simulink model "OFDM_8_Point"  (R2022a)
settings: Solver=VariableStepAuto  StartTime=0.0  StopTime=1000  RelTol=1e-3
undefined symbols (not defined in the file): xc7s100fgga676
libraries: hdlBasic x39, commrandsrc3 x1, vmcUtilities x1
settings Model: Creator=Sandesh  LastModifiedBy=Sandesh

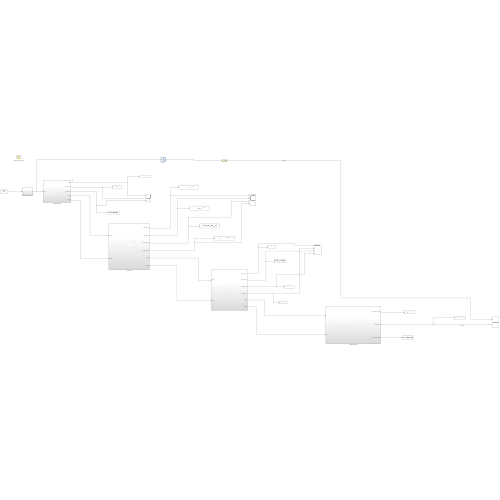
[thumbnail: Simulink's stored preview of the top-level diagram]
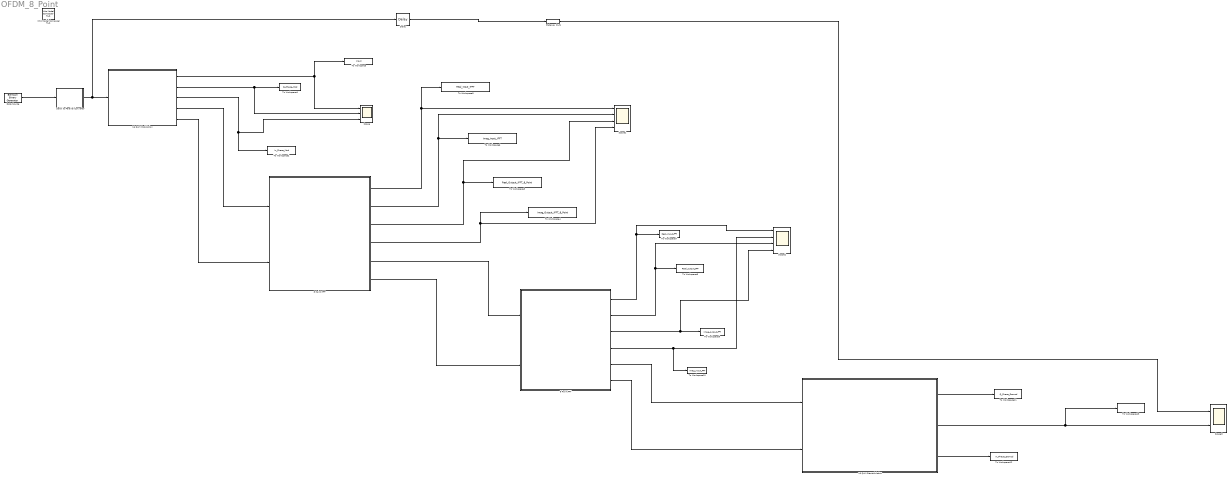
== system OFDM_8_Point ==
  16 QAM Demodulation : Subsystem
  16 QAM Modulation : Subsystem
  8 Point FFT : Subsystem
  8 Point IFFT : Subsystem
  Data Source : commrandsrc3/Bernoulli Binary Generator  ProbabilityOfZero=0.5  SeedSource=Auto  Seed=0  SampleTime=1  SamplesPerFrame=1  OutputDataType=double  SimulateUsing=Interpreted execution
  Delay : hdlBasic/Delay  rst=off  en=off  latency=129  reg_retiming=off  XmcBlockStatus=1  maskContainerNames=group1  block_type=delay  block_config=sysgen:Delay_config
  Gateway Out1 : hdlBasic/Gateway Out  inherit_from_input=off  hdl_port=on  rows=1  columns=1  UseAsDAC=off  DACChannel='1'  interface=None  automatic_assignment=on  address_offset=hex2dec('00')  intf_name=''  intf_description=''  timing_constraint=None  locs_specified=off  LOCs={}  io_standard={}  XmcBlockStatus=1  maskContainerNames=group4  block_type=gatewayout  block_config=sysgen:gateway_out_config  block_width_w=590  block_height_w=620  block_width=620  block_height=750
  Scope : Scope  NumInputPorts=3
  Scope1 : Scope  NumInputPorts=4
  Scope2 : Scope  NumInputPorts=4
  Scope3 : Scope  NumInputPorts=2
  Serial to Parallel Converter : Subsystem
  To Workspace : ToWorkspace  VariableName=Input  SaveFormat=Timeseries  SampleTime=-1
  To Workspace1 : ToWorkspace  VariableName=Q_Phase_Mod  SaveFormat=Timeseries  SampleTime=-1
  To Workspace10 : ToWorkspace  VariableName=Imag_Input_FFT  SaveFormat=Timeseries  SampleTime=-1
  To Workspace11 : ToWorkspace  VariableName=Q_Phase_Demod  SaveFormat=Timeseries  SampleTime=-1
  To Workspace12 : ToWorkspace  VariableName=In_Phase_Demod  SaveFormat=Timeseries  SampleTime=-1
  To Workspace13 : ToWorkspace  VariableName=Output_after_demodulation  SaveFormat=Timeseries  SampleTime=-1
  To Workspace2 : ToWorkspace  VariableName=In_Phase_Mod  SaveFormat=Timeseries  SampleTime=-1
  To Workspace3 : ToWorkspace  VariableName=Real_Output_IFFT_8_Point  SaveFormat=Timeseries  SampleTime=-1
  To Workspace4 : ToWorkspace  VariableName=Imag_Output_IFFT_8_Point  SaveFormat=Timeseries  SampleTime=-1
  To Workspace5 : ToWorkspace  VariableName=Real_Input_IFFT  SaveFormat=Timeseries  SampleTime=-1
  To Workspace6 : ToWorkspace  VariableName=Imag_Input_IFFT  SaveFormat=Timeseries  SampleTime=-1
  To Workspace7 : ToWorkspace  VariableName=Real_Input_FFT  SaveFormat=Timeseries  SampleTime=-1
  To Workspace8 : ToWorkspace  VariableName=Real_output_FFT  SaveFormat=Timeseries  SampleTime=-1
  To Workspace9 : ToWorkspace  VariableName=Imag_output_FFT  SaveFormat=Timeseries  SampleTime=-1
  Vitis Model Composer Hub : vmcUtilities/Vitis Model Composer Hub  Tag=genX  CodeGeneration=off  TargetDirectory=./code  ExportType=AI Engines  IpVendor=xilinx.com  IpLibrary=hls  IpVersion=1.0  IpHWLanguage=Verilog  AieCompilerOptions={}  CreateTestbench=off  TestbenchStackSize=10  RunAieSim=off  AieSimTimeout=50000  RunAieSimProfiling=off  LaunchVitisAnalyzer=off  PlotOutput=off  RunX86Sim=off  X86SimTimeout=10  GenHwImage=off  PlatformType=Not Specified  HwSystemType=Baremetal  HwValidationTarget=hw  ProjDevice=Spartan-7 SP701 Evaluation Platform (xc7s100fgga676-2)  ProjDevicePart=xc7s100fgga676-2  SamplePeriod=-1  ClockFrequency=200  DataPathParallelism=1  xilinxfamily=spartan7  part=xc7s100  speed=-2  package=fgga676  directory=./netlist  testbench=on  incr_netlist=off  synthesis_tool=Vivado  clock_wrapper=Clock Enables  dbl_ovrd=According to Block Masks  dcm_input_clock_period=10  sysclk_period=10  simulink_period=1  eval_field=0  IPInfoJsonString="{\"HDLSubsystem\":{\"SubsystemName\":\"QAM_16_Point\",\"IPName\":\"QAM_16_Point\",\"IPLibrary\":\"VMC\",\"IPVendor\":\"User Company\",\"IPVersion\":\"1.0\"}}"
  wires:
  Data Source/1 -> Serial to Parallel Converter/1(S)
  8 Point IFFT/4(Imag_Output_IFFT) -> Scope1/4, To Workspace4/1
  8 Point IFFT/3(Real_Output_IFFT) -> Scope1/3, To Workspace3/1
  8 Point IFFT/2(Imag_Input_IFFT) -> Scope1/2, To Workspace6/1
  8 Point IFFT/1(Real_Input_IFFT) -> Scope1/1, To Workspace5/1
  8 Point FFT/2(Real_Output_FFT) -> Scope2/3, To Workspace8/1
  8 Point FFT/3(Imag_Output_FFT) -> To Workspace9/1, Scope2/4
  8 Point FFT/1(Real_Input_FFT) -> Scope2/1, To Workspace7/1
  8 Point FFT/4(Imag_Input_FFT) -> Scope2/2, To Workspace10/1
  8 Point IFFT/5(Real_Out) -> 8 Point FFT/1(In_Real)
  8 Point IFFT/6(Imag_Out) -> 8 Point FFT/2(In_Imag)
  Delay/1 -> Gateway Out1/1
  Gateway Out1/1 -> Scope3/1  "Initial_Input"
  16 QAM Demodulation/2(DeMod_Output) -> Scope3/2, To Workspace13/1  "Final_Output"
  8 Point FFT/5(Imag_out) -> 16 QAM Demodulation/1(Q_Phase)
  8 Point FFT/6(Real_out) -> 16 QAM Demodulation/2(In_Phase)
  16 QAM Demodulation/1(Q_Phase_Dmod_Output) -> To Workspace11/1
  16 QAM Demodulation/3(In_Phase_Dmod_Output) -> To Workspace12/1
  Serial to Parallel Converter/1(P) -> 16 QAM Modulation/1(In_4_bit), Delay/1
  16 QAM Modulation/1(Input) -> Scope/1, To Workspace/1
  16 QAM Modulation/3(In_Phase_Mod1) -> Scope/3, To Workspace2/1
  16 QAM Modulation/2(Q_Phase_Mod1) -> Scope/2, To Workspace1/1
  16 QAM Modulation/4(Real_In) -> 8 Point IFFT/1(In_Real)
  16 QAM Modulation/5(Imag_In) -> 8 Point IFFT/2(In_Imag)

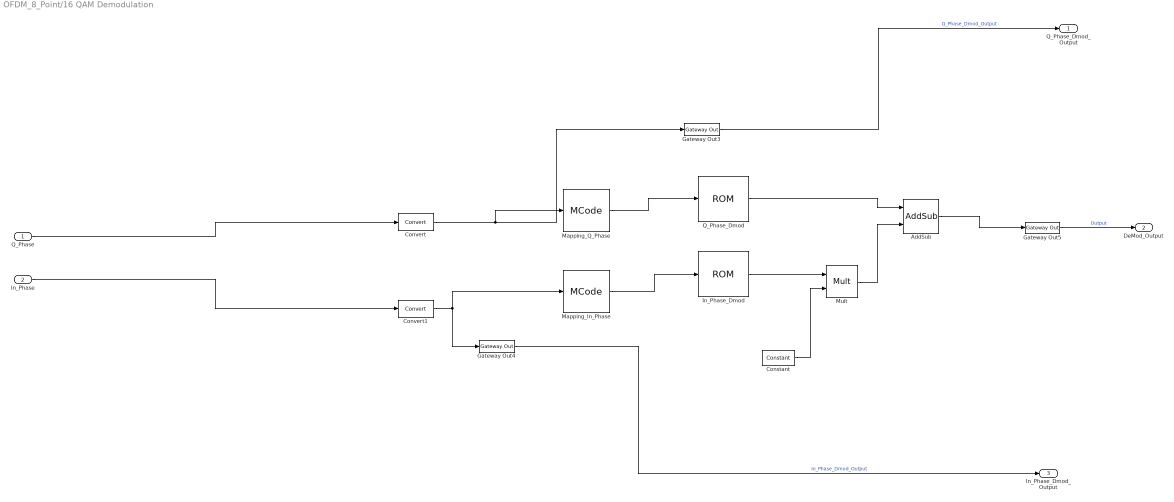
== system OFDM_8_Point/16 QAM Demodulation ==
  Q_Phase : Inport
  In_Phase : Inport  Port=2
  AddSub : hdlBasic/AddSub  mode=Addition  use_carryin=off  use_carryout=off  en=off  latency=0  precision=Full  arith_type=Unsigned  n_bits=16  bin_pt=14  quantization=Truncate  overflow=Wrap  use_behavioral_HDL=off  hw_selection=Fabric  pipelined=off  XmcBlockStatus=1  maskContainerNames=tabcontainer1  block_type=addsub  block_config=sysgen:Addsub_config
  Constant : hdlBasic/Constant  const=4  gui_display_data_type=Fixed-point  arith_type=Unsigned  n_bits=4  bin_pt=0  preci_type=Single  exp_width=8  frac_width=24  explicit_period=off  period=1  XmcBlockStatus=1  maskContainerNames=tabcontainer1  block_type=constant  block_config=sysgen:Constant_config
  Convert : hdlBasic/Convert  gui_display_data_type=Fixed-point  arith_type=Signed (2's comp)  n_bits=30  bin_pt=10  float_type=Single  exp_bits=8  fraction_bits=24  quantization="Round  (unbiased: +/- Inf)"  overflow=Wrap  en=off  latency=1  pipeline=off  XmcBlockStatus=1  maskContainerNames=group2  block_type=convert  block_config=sysgen:Convert_config  block_width=595  block_height=885
  Convert1 : hdlBasic/Convert  gui_display_data_type=Fixed-point  arith_type=Signed (2's comp)  n_bits=30  bin_pt=10  float_type=Single  exp_bits=8  fraction_bits=24  quantization="Round  (unbiased: +/- Inf)"  overflow=Wrap  en=off  latency=1  pipeline=off  XmcBlockStatus=1  maskContainerNames=group2  block_type=convert  block_config=sysgen:Convert_config  block_width=595  block_height=885
  Gateway Out3 : hdlBasic/Gateway Out  inherit_from_input=off  hdl_port=on  rows=1  columns=1  UseAsDAC=off  DACChannel='1'  interface=None  automatic_assignment=on  address_offset=hex2dec('00')  intf_name=''  intf_description=''  timing_constraint=None  locs_specified=off  LOCs={}  io_standard={}  XmcBlockStatus=1  maskContainerNames=group4  block_type=gatewayout  block_config=sysgen:gateway_out_config  block_width_w=590  block_height_w=620  block_width=620  block_height=750
  Gateway Out4 : hdlBasic/Gateway Out  inherit_from_input=off  hdl_port=on  rows=1  columns=1  UseAsDAC=off  DACChannel='1'  interface=None  automatic_assignment=on  address_offset=hex2dec('00')  intf_name=''  intf_description=''  timing_constraint=None  locs_specified=off  LOCs={}  io_standard={}  XmcBlockStatus=1  maskContainerNames=group4  block_type=gatewayout  block_config=sysgen:gateway_out_config  block_width_w=590  block_height_w=620  block_width=620  block_height=750
  Gateway Out5 : hdlBasic/Gateway Out  inherit_from_input=off  hdl_port=on  rows=1  columns=1  UseAsDAC=off  DACChannel='1'  interface=None  automatic_assignment=on  address_offset=hex2dec('00')  intf_name=''  intf_description=''  timing_constraint=None  locs_specified=off  LOCs={}  io_standard={}  XmcBlockStatus=1  maskContainerNames=group4  block_type=gatewayout  block_config=sysgen:gateway_out_config  block_width_w=590  block_height_w=620  block_width=620  block_height=750
  In_Phase_Dmod : hdlBasic/ROM  depth=4  initVector=[0 1 2 3]  distributed_mem=Block RAM  rst=off  init_reg=0  en=off  latency=1  gui_display_data_type=Fixed-point  arith_type=Unsigned  n_bits=2  bin_pt=0  preci_type=Double  exp_width=8  frac_width=24  optimize=Area  use_rpm=on  simulation_type=fast_sim  XmcBlockStatus=1  maskContainerNames=tabcontainer1  block_type=sprom  block_config=sysgen:SPROM_config
  Mapping_In_Phase : hdlBasic/MCode  mfname=Mapping  explicit_period=off  period=1  iptable={ 'I', '' }  optable={ 'B', 'off' }  enable_stdout=off  enable_debug=off  suppress_output='on'  defparams={}  hide_port_list={}  block_type=mcode  block_width=444  block_height=788
      settings: infoedit=Pass input values to a MATLAB function for evaluation in Xilinx fixed-point type. The input ports of the block are input arguments of the function. The output ports of the block are output arguments of the function.
  Mapping_Q_Phase : hdlBasic/MCode  mfname=Mapping  explicit_period=off  period=1  iptable={ 'I', '' }  optable={ 'B', 'off' }  enable_stdout=off  enable_debug=off  suppress_output='on'  defparams={}  hide_port_list={}  block_type=mcode  block_width=444  block_height=788
      settings: infoedit=Pass input values to a MATLAB function for evaluation in Xilinx fixed-point type. The input ports of the block are input arguments of the function. The output ports of the block are output arguments of the function.
  Mult : hdlBasic/Mult  precision=Full  arith_type=Unsigned  n_bits=4  bin_pt=14  quantization=Truncate  overflow=Wrap  en=off  latency=0  use_behavioral_HDL=off  opt=Speed  use_embedded=on  optimum_pipeline=off  pipeline=on  use_rpm=on  placement_style=Triangular  XmcBlockStatus=1  maskContainerNames=group1  block_type=mult  block_config=sysgen:Mult_config  block_width=598  block_height=876
  Q_Phase_Dmod : hdlBasic/ROM  depth=4  initVector=[3 2 1 0]  distributed_mem=Block RAM  rst=off  init_reg=0  en=off  latency=1  gui_display_data_type=Fixed-point  arith_type=Unsigned  n_bits=2  bin_pt=0  preci_type=Double  exp_width=8  frac_width=24  optimize=Area  use_rpm=on  simulation_type=fast_sim  XmcBlockStatus=1  maskContainerNames=tabcontainer1  block_type=sprom  block_config=sysgen:SPROM_config
  Q_Phase_Dmod_Output : Outport
  DeMod_Output : Outport  Port=2
  In_Phase_Dmod_Output : Outport  Port=3
  wires:
  Constant/1 -> Mult/2
  Convert1/1 -> Mapping_In_Phase/1, Gateway Out4/1
  AddSub/1 -> Gateway Out5/1
  Mapping_Q_Phase/1 -> Q_Phase_Dmod/1
  Q_Phase_Dmod/1 -> AddSub/1
  In_Phase_Dmod/1 -> Mult/1
  Convert/1 -> Gateway Out3/1, Mapping_Q_Phase/1
  Mapping_In_Phase/1 -> In_Phase_Dmod/1
  Mult/1 -> AddSub/2
  Gateway Out5/1 -> DeMod_Output/1  "Output"
  Q_Phase/1 -> Convert/1
  Gateway Out3/1 -> Q_Phase_Dmod_Output/1  "Q_Phase_Dmod_Output"
  In_Phase/1 -> Convert1/1
  Gateway Out4/1 -> In_Phase_Dmod_Output/1  "In_Phase_Dmod_Output"

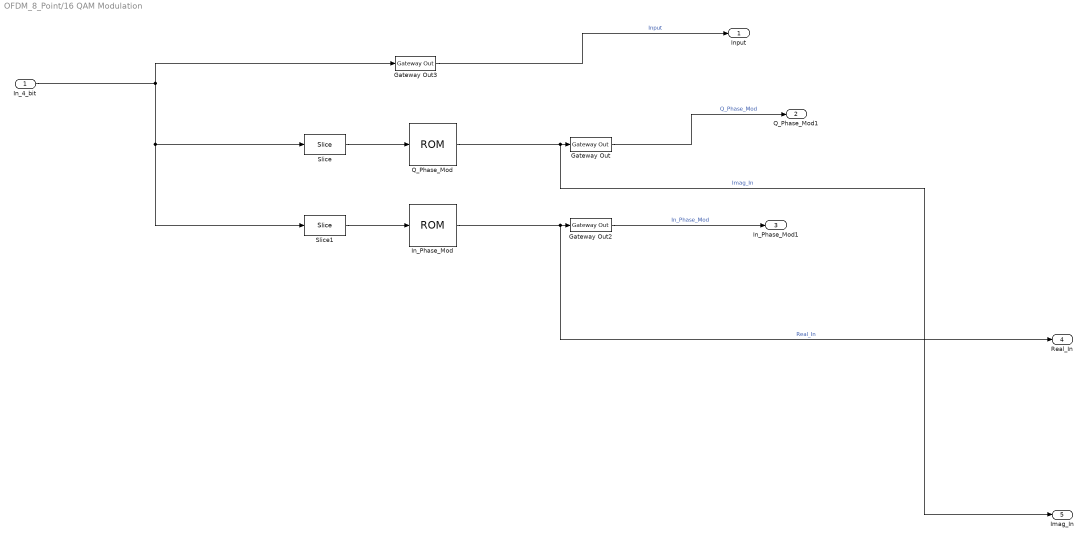
== system OFDM_8_Point/16 QAM Modulation ==
  In_4_bit : Inport
  Gateway Out : hdlBasic/Gateway Out  inherit_from_input=off  hdl_port=on  rows=1  columns=1  UseAsDAC=off  DACChannel='1'  interface=None  automatic_assignment=on  address_offset=hex2dec('00')  intf_name=''  intf_description=''  timing_constraint=None  locs_specified=off  LOCs={}  io_standard={}  XmcBlockStatus=1  maskContainerNames=group4  block_type=gatewayout  block_config=sysgen:gateway_out_config  block_width_w=590  block_height_w=620  block_width=620  block_height=750
  Gateway Out2 : hdlBasic/Gateway Out  inherit_from_input=off  hdl_port=on  rows=1  columns=1  UseAsDAC=off  DACChannel='1'  interface=None  automatic_assignment=on  address_offset=hex2dec('00')  intf_name=''  intf_description=''  timing_constraint=None  locs_specified=off  LOCs={}  io_standard={}  XmcBlockStatus=1  maskContainerNames=group4  block_type=gatewayout  block_config=sysgen:gateway_out_config  block_width_w=590  block_height_w=620  block_width=620  block_height=750
  Gateway Out3 : hdlBasic/Gateway Out  inherit_from_input=off  hdl_port=on  rows=1  columns=1  UseAsDAC=off  DACChannel='1'  interface=None  automatic_assignment=on  address_offset=hex2dec('00')  intf_name=''  intf_description=''  timing_constraint=None  locs_specified=off  LOCs={}  io_standard={}  XmcBlockStatus=1  maskContainerNames=group4  block_type=gatewayout  block_config=sysgen:gateway_out_config  block_width_w=590  block_height_w=620  block_width=620  block_height=750
  In_Phase_Mod : hdlBasic/ROM  depth=4  initVector=[-3 -1 +1 +3]  distributed_mem=Block RAM  rst=off  init_reg=0  en=off  latency=1  gui_display_data_type=Fixed-point  arith_type="Signed  (2's comp)"  n_bits=16  bin_pt=13  preci_type=Single  exp_width=8  frac_width=24  optimize=Area  use_rpm=on  simulation_type=fast_sim  XmcBlockStatus=1  maskContainerNames=tabcontainer1  block_type=sprom  block_config=sysgen:SPROM_config
  Q_Phase_Mod : hdlBasic/ROM  depth=4  initVector=[+3 +1 -1 -3]  distributed_mem=Block RAM  rst=off  init_reg=0  en=off  latency=1  gui_display_data_type=Fixed-point  arith_type="Signed  (2's comp)"  n_bits=16  bin_pt=13  preci_type=Single  exp_width=8  frac_width=24  optimize=Area  use_rpm=on  simulation_type=fast_sim  XmcBlockStatus=1  maskContainerNames=tabcontainer1  block_type=sprom  block_config=sysgen:SPROM_config
  Slice : hdlBasic/Slice  nbits=2  boolean_output=off  mode=Lower Bit Location + Width  bit1=0  base1=MSB of Input  bit0=0  base0=LSB of Input  XmcBlockStatus=1  maskContainerNames=group1  block_type=slice  block_config=sysgen:Slice_config
  Slice1 : hdlBasic/Slice  nbits=2  boolean_output=off  mode=Upper Bit Location + Width  bit1=0  base1=MSB of Input  bit0=0  base0=LSB of Input  XmcBlockStatus=1  maskContainerNames=group1  block_type=slice  block_config=sysgen:Slice_config
  Input : Outport
  Q_Phase_Mod1 : Outport  Port=2
  In_Phase_Mod1 : Outport  Port=3
  Real_In : Outport  Port=4
  Imag_In : Outport  Port=5
  wires:
  Gateway Out2/1 -> In_Phase_Mod1/1  "In_Phase_Mod"
  Slice/1 -> Q_Phase_Mod/1
  In_4_bit/1 -> Slice1/1, Slice/1, Gateway Out3/1
  In_Phase_Mod/1 -> Real_In/1, Gateway Out2/1  "Real_In"
  Q_Phase_Mod/1 -> Imag_In/1, Gateway Out/1  "Imag_In"
  Slice1/1 -> In_Phase_Mod/1
  Gateway Out3/1 -> Input/1  "Input"
  Gateway Out/1 -> Q_Phase_Mod1/1  "Q_Phase_Mod"

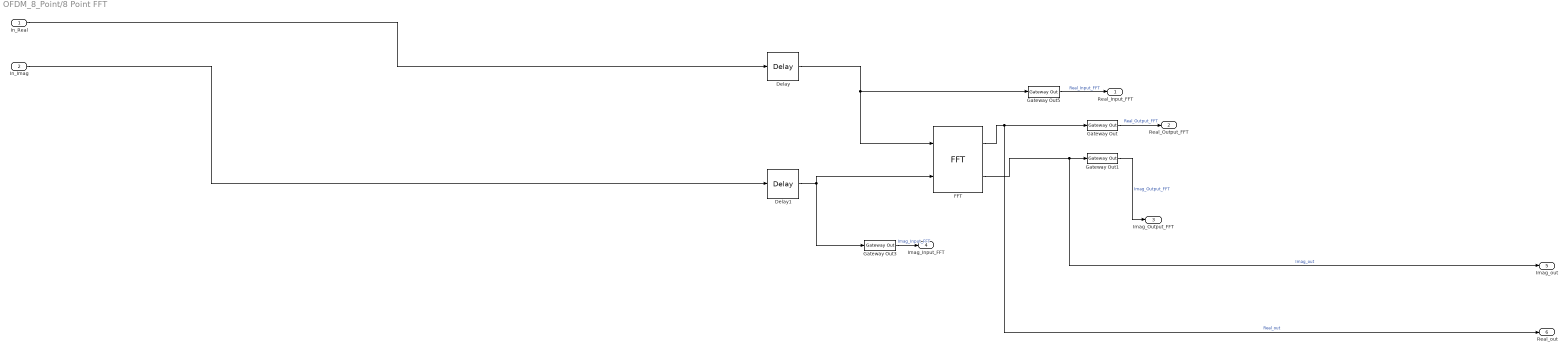
== system OFDM_8_Point/8 Point FFT ==
  In_Real : Inport
  In_Imag : Inport  Port=2
  Delay : hdlBasic/Delay  rst=off  en=off  latency=3  reg_retiming=off  XmcBlockStatus=1  maskContainerNames=group1  block_type=delay  block_config=sysgen:Delay_config
  Delay1 : hdlBasic/Delay  rst=off  en=off  latency=3  reg_retiming=off  XmcBlockStatus=1  maskContainerNames=group1  block_type=delay  block_config=sysgen:Delay_config
  FFT : hdlBasic/FFT  transform_length=8  scale_result_by_fft_length=off  bit_reversed_order=on  optimizegoal=Performance  start_frame=off  simulation_type=fast_sim  simulation_model=sysgen:ForwardFFT_Macro  latency=1  XmcBlockStatus=1  maskContainerNames=group1  block_type=xfft_forward  block_config=sysgen:FFTMacro_config
  Gateway Out{,1,3,5} (4 alike) : hdlBasic/Gateway Out  inherit_from_input=off  hdl_port=on  rows=1  columns=1  UseAsDAC=off  DACChannel='1'  interface=None  automatic_assignment=on  address_offset=hex2dec('00')  intf_name=''  intf_description=''  timing_constraint=None  locs_specified=off  LOCs={}  io_standard={}  XmcBlockStatus=1  maskContainerNames=group4  block_type=gatewayout  block_config=sysgen:gateway_out_config  block_width_w=590  block_height_w=620  block_width=620  block_height=750
  Real_Input_FFT : Outport
  Real_Output_FFT : Outport  Port=2
  Imag_Output_FFT : Outport  Port=3
  Imag_Input_FFT : Outport  Port=4
  Imag_out : Outport  Port=5
  Real_out : Outport  Port=6
  wires:
  FFT/1 -> Real_out/1, Gateway Out/1  "Real_out"
  FFT/2 -> Imag_out/1, Gateway Out1/1  "Imag_out"
  Gateway Out3/1 -> Imag_Input_FFT/1  "Imag_Input_FFT"
  Delay1/1 -> FFT/2, Gateway Out3/1
  Delay/1 -> FFT/1, Gateway Out5/1
  Gateway Out/1 -> Real_Output_FFT/1  "Real_Output_FFT"
  Gateway Out5/1 -> Real_Input_FFT/1  "Real_Input_FFT"
  Gateway Out1/1 -> Imag_Output_FFT/1  "Imag_Output_FFT"
  In_Imag/1 -> Delay1/1
  In_Real/1 -> Delay/1

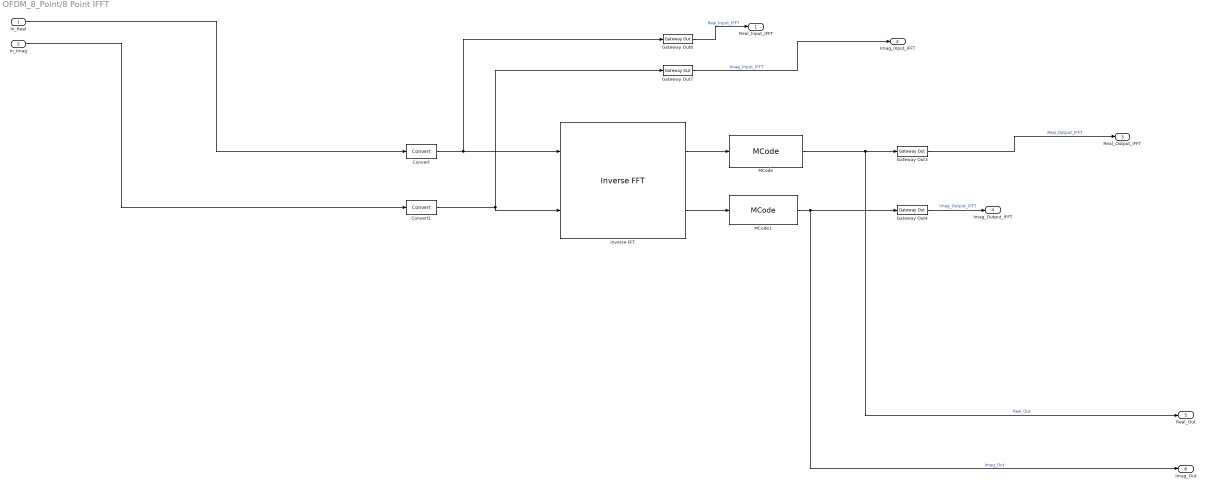
== system OFDM_8_Point/8 Point IFFT ==
  In_Real : Inport
  In_Imag : Inport  Port=2
  Convert : hdlBasic/Convert  gui_display_data_type=Fixed-point  arith_type=Signed (2's comp)  n_bits=30  bin_pt=10  float_type=Single  exp_bits=8  fraction_bits=24  quantization=Truncate  overflow=Wrap  en=off  latency=1  pipeline=off  XmcBlockStatus=1  maskContainerNames=group2  block_type=convert  block_config=sysgen:Convert_config  block_width=595  block_height=885
  Convert1 : hdlBasic/Convert  gui_display_data_type=Fixed-point  arith_type=Signed (2's comp)  n_bits=30  bin_pt=10  float_type=Single  exp_bits=8  fraction_bits=24  quantization=Truncate  overflow=Wrap  en=off  latency=1  pipeline=off  XmcBlockStatus=1  maskContainerNames=group2  block_type=convert  block_config=sysgen:Convert_config  block_width=595  block_height=885
  Gateway Out{3..4,6..7} (4 alike) : hdlBasic/Gateway Out  inherit_from_input=off  hdl_port=on  rows=1  columns=1  UseAsDAC=off  DACChannel='1'  interface=None  automatic_assignment=on  address_offset=hex2dec('00')  intf_name=''  intf_description=''  timing_constraint=None  locs_specified=off  LOCs={}  io_standard={}  XmcBlockStatus=1  maskContainerNames=group4  block_type=gatewayout  block_config=sysgen:gateway_out_config  block_width_w=590  block_height_w=620  block_width=620  block_height=750
  Inverse FFT : hdlBasic/Inverse FFT  transform_length=8  scale_result_by_fft_length=off  bit_reversed_order=on  optimizegoal=Performance  start_frame=off  simulation_type=fast_sim  simulation_model=sysgen:InverseFFT_Macro  latency=1  XmcBlockStatus=1  maskContainerNames=group1  block_type=xfft_inverse  block_config=sysgen:Inverse_FFTMacro_config
  MCode : hdlBasic/MCode  mfname=divideby8  explicit_period=off  period=1  iptable={ 'A', '' }  optable={ 'B', 'off' }  enable_stdout=off  enable_debug=off  suppress_output='on'  defparams={}  hide_port_list={}  block_type=mcode  block_width=444  block_height=788
      settings: infoedit=Pass input values to a MATLAB function for evaluation in Xilinx fixed-point type. The input ports of the block are input arguments of the function. The output ports of the block are output arguments of the function.
  MCode1 : hdlBasic/MCode  mfname=divideby8  explicit_period=off  period=1  iptable={ 'A', '' }  optable={ 'B', 'off' }  enable_stdout=off  enable_debug=off  suppress_output='on'  defparams={}  hide_port_list={}  block_type=mcode  block_width=444  block_height=788
      settings: infoedit=Pass input values to a MATLAB function for evaluation in Xilinx fixed-point type. The input ports of the block are input arguments of the function. The output ports of the block are output arguments of the function.
  Real_Input_IFFT : Outport
  Imag_Input_IFFT : Outport  Port=2
  Real_Output_IFFT : Outport  Port=3
  Imag_Output_IFFT : Outport  Port=4
  Real_Out : Outport  Port=5
  Imag_Out : Outport  Port=6
  wires:
  Inverse FFT/2 -> MCode1/1
  MCode1/1 -> Imag_Out/1, Gateway Out4/1  "Imag_Out"
  MCode/1 -> Real_Out/1, Gateway Out3/1  "Real_Out"
  Convert/1 -> Gateway Out6/1, Inverse FFT/1
  Inverse FFT/1 -> MCode/1
  Convert1/1 -> Inverse FFT/2, Gateway Out7/1
  Gateway Out3/1 -> Real_Output_IFFT/1  "Real_Output_IFFT"
  Gateway Out7/1 -> Imag_Input_IFFT/1  "Imag_Input_IFFT"
  Gateway Out6/1 -> Real_Input_IFFT/1  "Real_Input_IFFT"
  Gateway Out4/1 -> Imag_Output_IFFT/1  "Imag_Output_IFFT"
  In_Real/1 -> Convert/1
  In_Imag/1 -> Convert1/1

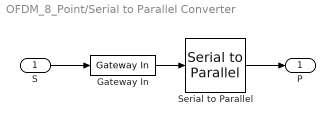
== system OFDM_8_Point/Serial to Parallel Converter ==
  S : Inport
  Gateway In : hdlBasic/Gateway In  gui_display_data_type=Fixed-point  arith_type=Unsigned  n_bits=1  bin_pt=0  preci_type=Single  exp_width=8  frac_width=24  rows=1  columns=1  quantization="Round  (unbiased: +/- Inf)"  overflow=Saturate  period=1  UseAsADC=off  ADCChannel='1'  interface=None  automatic_assignment=on  address_offset=hex2dec('00')  intf_name=''  intf_description=''  default_value=0  timing_constraint=None  locs_specified=off  LOCs={}  io_standard={}  inherit_from_input=off  hdl_port=on  XmcBlockStatus=1  maskContainerNames=group4  block_type=gatewayin  block_config=sysgen:gateway_in_config  block_width_w=590  block_height_w=620  block_width=640  block_height=850
  Serial to Parallel : hdlBasic/Serial to Parallel  input_order=Least Significant Word First  arith_type=Unsigned  output_bits=4  bin_pt=0  rst=off  en=off  latency=1  input_bits=[]  XmcBlockStatus=1  maskContainerNames=group3  block_type=s2p  block_config=sysgen:S2P_config
  P : Outport
  wires:
  Gateway In/1 -> Serial to Parallel/1
  S/1 -> Gateway In/1
  Serial to Parallel/1 -> P/1
